simulink model "kinematik_simulation"  (R2020a)
settings: Solver=VariableStepAuto  StartTime=0.0  StopTime=10.0  RelTol=1e-3
values from neighbouring files (symbols this model uses):
  d = 5    [konstanten.m]
  g = 9.8    [konstanten.m]
  J = 1500    [konstanten.m]
  l = 0.2    [konstanten.m]
  m = 0.03    [konstanten.m]
settings Model: Creator=junio  LastModifiedBy=junio

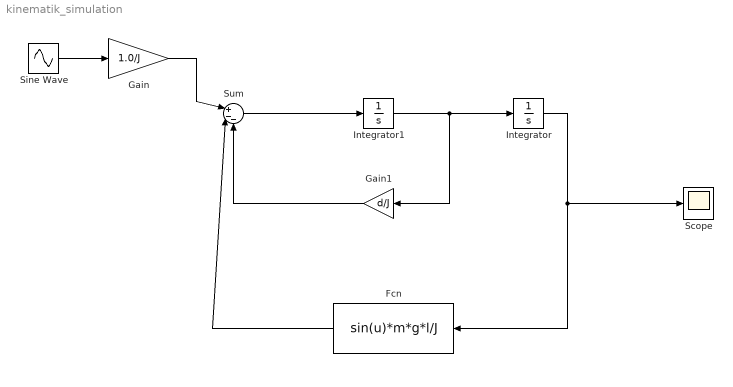
== system kinematik_simulation ==
  Fcn : Fcn  Expr=sin(u)*m*g*l/J
  Gain : Gain  Gain=1.0/J
  Gain1 : Gain  Gain=d/J
  Integrator : Integrator
  Integrator1 : Integrator
  Scope : Scope
  Sine Wave : Sin  SampleTime=0
  Sum : Sum  Inputs=|+--
  wires:
  Sine Wave/1 -> Gain/1
  Gain/1 -> Sum/1
  Sum/1 -> Integrator1/1
  Gain1/1 -> Sum/3
  Fcn/1 -> Sum/2
  Integrator1/1 -> Integrator/1, Gain1/1
  Integrator/1 -> Scope/1, Fcn/1
